simulink model "task_4_scheme"  (R2024a)
settings: Solver=FixedStepAuto  StartTime=0.0  StopTime=15.0  FixedStep=1e-4  RelTol=1e-3
settings Model: Creator=alexe  LastModifiedBy=alexe

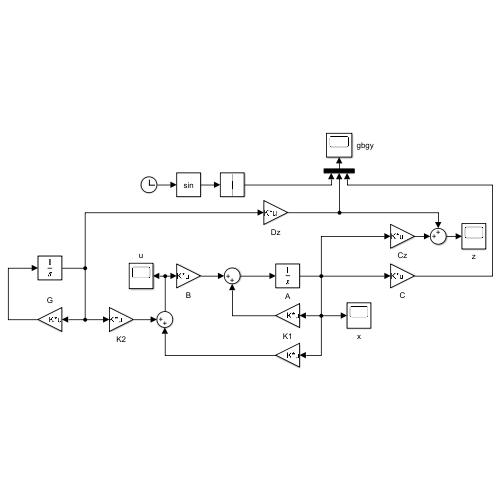
[thumbnail: Simulink's stored preview of the top-level diagram]
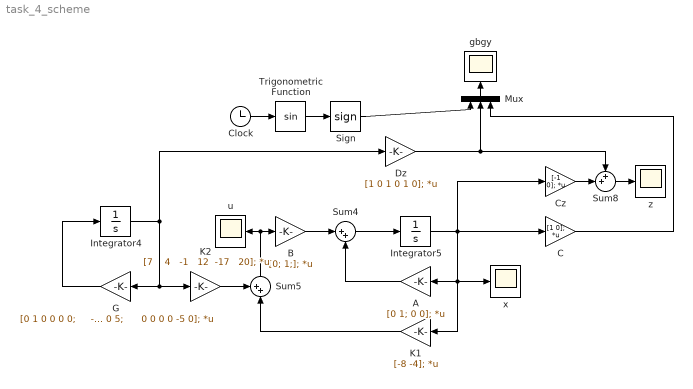
== system task_4_scheme ==
  A : Gain  Gain=[0 1; 0 0];  Multiplication=Matrix(K*u)
  B : Gain  Gain=[0; 1;];  Multiplication=Matrix(K*u)
  C : Gain  Gain=[1 0];  Multiplication=Matrix(K*u)
  Clock : Clock
  Cz : Gain  Gain=[-1 0];  Multiplication=Matrix(K*u)
  Dz : Gain  Gain=[1 0 1 0 1 0];  Multiplication=Matrix(K*u)
  G : Gain  Gain=|  Multiplication=Matrix(K*u)
      | [0 1 0 0 0 0;
      |     -1 0 0 0 0 0;
      |      0 0 0 3 0 0;
      |      0 0 -3 0 0 0;
      |      0 0 0 0 0 5;
      |      0 0 0 0 -5 0];
  Integrator4 : Integrator  InitialCondition=[0;4/pi;0;4/(3*pi);0;4/(5*pi)];
  Integrator5 : Integrator  InitialCondition=[0;0]
  K1 : Gain  Gain=[-8 -4];  Multiplication=Matrix(K*u)
  K2 : Gain  Gain="[7    4   -1   12  -17   20];"  Multiplication=Matrix(K*u)
  Mux : Mux  Inputs=3
  Sign : Signum
  Sum4 : Sum  Inputs=|++
  Sum5 : Sum  Inputs=++|
  Sum8 : Sum  Inputs=++|
  Trigonometric Function : Trigonometry
  gbgy : Scope
  u : Scope
  x : Scope
  z : Scope
  wires:
  K1/1 -> Sum5/2
  Integrator4/1 -> Dz/1, K2/1, G/1
  Sum5/1 -> u/1, B/1
  Integrator5/1 -> C/1, Cz/1, x/1, K1/1, A/1
  Sum4/1 -> Integrator5/1
  G/1 -> Integrator4/1
  K2/1 -> Sum5/1
  A/1 -> Sum4/2
  B/1 -> Sum4/1
  Cz/1 -> Sum8/2
  Sum8/1 -> z/1
  Dz/1 -> Sum8/1, Mux/2
  Clock/1 -> Trigonometric Function/1
  Trigonometric Function/1 -> Sign/1
  Mux/1 -> gbgy/1
  C/1 -> Mux/3
  Sign/1 -> Mux/1
